simulink model "full_correlator"  (R2022a)
settings: Solver=VariableStepDiscrete  StartTime=0.0  StopTime=4000  RelTol=1e-3
libraries: hdlBasic x2638, hdlSSR x215, hdlDSPIP x4, xbsIndex_r4 x1, xps_library x1
(part 6 of 43)

== system full_correlator/Subsystem2/shared_bram3 ==
  addr : Inport
  data_in : Inport  Port=2
  we : Inport  Port=3
  Terminator : Terminator
  Terminator1 : Terminator
  Terminator2 : Terminator
  calc_add : Subsystem  mask{data_width=128, addr_width=6, sample_rate=sample_rate}
      mask prompts: data_width "data width"; addr_width "address width"; sample_rate "sample rate"
  convert_addr : hdlBasic/Convert  gui_display_data_type=Fixed-point  arith_type=Unsigned  n_bits=addr_width  bin_pt=0  float_type=Single  exp_bits=8  fraction_bits=24  quantization=Truncate  overflow=Wrap  en=off  latency=0  pipeline=off  XmcBlockStatus=1  maskContainerNames=group2  block_type=convert  block_config=sysgen:Convert_config  block_width=595  block_height=885
  convert_din1 : hdlBasic/Convert  gui_display_data_type=Fixed-point  arith_type=Unsigned  n_bits=128  bin_pt=0  float_type=Single  exp_bits=8  fraction_bits=24  quantization=Truncate  overflow=Wrap  en=off  latency=0  pipeline=off  XmcBlockStatus=1  maskContainerNames=group2  block_type=convert  block_config=sysgen:Convert_config  block_width=595  block_height=885
  convert_we : hdlBasic/Convert  gui_display_data_type=Fixed-point  arith_type=Unsigned  n_bits=1  bin_pt=0  float_type=Single  exp_bits=8  fraction_bits=24  quantization=Truncate  overflow=Wrap  en=off  latency=0  pipeline=off  XmcBlockStatus=1  maskContainerNames=group2  block_type=convert  block_config=sysgen:Convert_config  block_width=595  block_height=885
  full_correlator_Subsystem2_shared_bram3_addr : hdlBasic/Gateway Out  inherit_from_input=off  hdl_port=on  rows=1  columns=1  UseAsDAC=off  DACChannel='1'  interface=None  automatic_assignment=on  address_offset=hex2dec('00')  intf_name=''  intf_description=''  timing_constraint=None  locs_specified=off  LOCs={'A5','B9','A9','C1','A3','G6','E9','A6','A7','A8','B8','B1','B3','D9','B5','B4','B6','C2'}  io_standard={}  XmcBlockStatus=1  maskContainerNames=group4  block_type=gatewayout  block_config=sysgen:gateway_out_config  block_width_w=590  block_height_w=620  block_width=620  block_height=750
      settings: sginterface={'Nallatech'=>{'xdspkit'=>{'non_memory_mapped_port'=>'uprev_Shared_BRAM_addr'}},'Xilinx'=>{'jtaghwcosim'=>{'non_memory_mapped_port'=>'uprev_Shared_BRAM_addr'},'xdspkit'=>{'non_memory_mapped_port'=>'uprev_Shared_BRAM_addr'}}}
  full_correlator_Subsystem2_shared_bram3_data_in : hdlBasic/Gateway Out  inherit_from_input=off  hdl_port=on  rows=1  columns=1  UseAsDAC=off  DACChannel='1'  interface=None  automatic_assignment=on  address_offset=hex2dec('00')  intf_name=''  intf_description=''  timing_constraint=None  locs_specified=off  LOCs={'B21','B22','A22','B23','B19','C19','A20','A21','A23','B24','A24','A25','E18','D18','C18','B18'}  io_standard={}  XmcBlockStatus=1  maskContainerNames=group4  block_type=gatewayout  block_config=sysgen:gateway_out_config  block_width_w=590  block_height_w=620  block_width=620  block_height=750
      settings: sginterface={'Nallatech'=>{'xdspkit'=>{'non_memory_mapped_port'=>'uprev_Shared_BRAM_data_in'}},'Xilinx'=>{'jtaghwcosim'=>{'non_memory_mapped_port'=>'uprev_Shared_BRAM_data_in'},'xdspkit'=>{'non_memory_mapped_port'=>'uprev_Shared_BRAM_data_in'}}}
  full_correlator_Subsystem2_shared_bram3_data_out : hdlBasic/Gateway In  gui_display_data_type=Fixed-point  arith_type=Unsigned  n_bits=128  bin_pt=0  preci_type=Single  exp_width=8  frac_width=24  rows=1  columns=1  quantization=Truncate  overflow=Wrap  period=sample_rate  UseAsADC=off  ADCChannel='1'  interface=None  automatic_assignment=on  address_offset=hex2dec('00')  intf_name=''  intf_description=''  default_value=0  timing_constraint=None  locs_specified=off  LOCs={}  io_standard={}  inherit_from_input=off  hdl_port=on  XmcBlockStatus=1  maskContainerNames=group4  block_type=gatewayin  block_config=sysgen:gateway_in_config  block_width_w=590  block_height_w=620  block_width=640  block_height=850
      settings: sginterface={'Nallatech'=>{'xdspkit'=>{'non_memory_mapped_port'=>'uprev_Shared_BRAM_data_out'}},'Xilinx'=>{'jtaghwcosim'=>{'non_memory_mapped_port'=>'uprev_Shared_BRAM_data_out'},'xdspkit'=>{'non_memory_mapped_port'=>'uprev_Shared_BRAM_data_out'}}}
  full_correlator_Subsystem2_shared_bram3_we : hdlBasic/Gateway Out  inherit_from_input=off  hdl_port=on  rows=1  columns=1  UseAsDAC=off  DACChannel='1'  interface=None  automatic_assignment=on  address_offset=hex2dec('00')  intf_name=''  intf_description=''  timing_constraint=None  locs_specified=off  LOCs={'A14'}  io_standard={}  XmcBlockStatus=1  maskContainerNames=group4  block_type=gatewayout  block_config=sysgen:gateway_out_config  block_width_w=590  block_height_w=620  block_width=620  block_height=750
  munge_in : Subsystem  AncestorBlock=casper_library_flow_control/munge  mask(munge){divisions=4, div_size=[32 32 32 32], order=[3  2  1  0], arith_type_out=Unsigned, bin_pt_out=0}
      mask prompts: divisions "Number of divisions"; div_size "Division size (bits)"; order "Division packing order"; arith_type_out "Output arithmetic type"; bin_pt_out "Output binary point"
      mask help: Splits an input bus into the specified number of divisions and then recombines them in the order specified (most significant division = 0,least = number divisions-1)
      mask init:
      | munge_init(gcb, ...
      |     'divisions', divisions, ...
      |     'div_size', div_size, ...
      |     'order', order, ...
      |     'arith_type_out', arith_type_out, ...
      |     'bin_pt_out', bin_pt_out);
      settings: AttributesFormatString=|
      | split:[32 32 32 32]
      | join:[3 2 1 0]
      | Unsigned [128,0]
      mask TypeOptions arith_type_out: Unsigned | Signed  (2's comp) | Floating-point
  munge_out : Subsystem  AncestorBlock=casper_library_flow_control/munge  mask(munge){divisions=4, div_size=[32 32 32 32], order=[3  2  1  0], arith_type_out=Unsigned, bin_pt_out=0}
      mask prompts: divisions "Number of divisions"; div_size "Division size (bits)"; order "Division packing order"; arith_type_out "Output arithmetic type"; bin_pt_out "Output binary point"
      mask help: Splits an input bus into the specified number of divisions and then recombines them in the order specified (most significant division = 0,least = number divisions-1)
      mask init:
      | munge_init(gcb, ...
      |     'divisions', divisions, ...
      |     'div_size', div_size, ...
      |     'order', order, ...
      |     'arith_type_out', arith_type_out, ...
      |     'bin_pt_out', bin_pt_out);
      settings: AttributesFormatString=|
      | split:[32 32 32 32]
      | join:[3 2 1 0]
      | Unsigned [128,0]
      mask TypeOptions arith_type_out: Unsigned | Signed  (2's comp) | Floating-point
  sim_mem : Subsystem  mask{arith_type=Unsigned, addr_width=6, data_width=128, data_bin_pt=0, init_vals=[0   1   2   3   4   5   6   7   8   9  10  11  12  13  14  15  16  17  18  19  20  21  22  23  24  25  26  27  28  29  30  31  32  33  34  35  36  37  38  39  40  41  42  43  44  45  46  47  48  49  50  51  52  53  54  55  56  57  58  59  60  61  62  63], sample_rate=1, csp_latency=1}
      mask prompts: arith_type "Output Data Type"; addr_width "Address width"; data_width "Data width"; data_bin_pt "Data Binary Point"; init_vals "Initial values"; sample_rate "Sample rate"; csp_latency "Latency"
      mask init:
      | % set_param([gcb, '/data_to_xilinx'], 'arith_type', arith_type)
      | % set_param([gcb, '/data_to_xilinx'], 'n_bits', get_param(gcb, 'data_width'))
      mask TypeOptions arith_type: Unsigned | Signed  (2's comp)
      mask TypeOptions data_width: 8 | 16 | 32 | 64 | 128
  data_out : Outport  VectorParamsAs1DForOutWhenUnconnected=off
  wires:
  munge_out/1(dout) -> data_out/1
  sim_mem/1(data_out) -> full_correlator_Subsystem2_shared_bram3_data_out/1
  full_correlator_Subsystem2_shared_bram3_data_out/1 -> munge_out/1(din)
  convert_addr/1 -> full_correlator_Subsystem2_shared_bram3_addr/1
  convert_din1/1 -> full_correlator_Subsystem2_shared_bram3_data_in/1
  data_in/1 -> munge_in/1(din)
  calc_add/1(out) -> convert_addr/1
  full_correlator_Subsystem2_shared_bram3_we/1 -> Terminator2/1
  full_correlator_Subsystem2_shared_bram3_data_in/1 -> Terminator1/1
  full_correlator_Subsystem2_shared_bram3_addr/1 -> Terminator/1
  convert_we/1 -> full_correlator_Subsystem2_shared_bram3_we/1
  addr/1 -> sim_mem/1(addr), calc_add/1(in)
  we/1 -> sim_mem/3(we), convert_we/1
  munge_in/1(dout) -> sim_mem/2(data), convert_din1/1

== system full_correlator/Subsystem5/Subsystem ==
  din : Inport
  hold : Inport  Port=2
  Concat : hdlBasic/Concat  num_inputs=2  XmcBlockStatus=1  maskContainerNames=group1  block_type=concat  block_config=sysgen:Concat_config
  Scalar to Vector : hdlSSR/Scalar2Vector  Width=18  sg_ssr=16  block_type=scalar2vector_ssr  XmcBlockStatus=1  sg_ssr_prev=16  maskContainerNames=group1
  Vector Register : hdlSSR/Vector Register  init=[0, 0, 0, 0, 0,0,0,0]  rst=off  en=on  sg_ssr=8  block_type=register_ssr  XmcBlockStatus=1  sg_ssr_prev=8  maskContainerNames=group2
  Vector Reinterpret : hdlSSR/Vector Reinterpret  force_arith_type=on  arith_type="Signed  (2's comp)"  force_bin_pt=on  bin_pt=17  sg_ssr=16  block_type=reinterpret_ssr  XmcBlockStatus=1  sg_ssr_prev=16  maskContainerNames=group1
  Vector Reinterpret1 : hdlSSR/Vector Reinterpret  force_arith_type=on  arith_type=Unsigned  force_bin_pt=on  bin_pt=0  sg_ssr=8  block_type=reinterpret_ssr  XmcBlockStatus=1  sg_ssr_prev=8  maskContainerNames=group1
  Vector Reinterpret2 : hdlSSR/Vector Reinterpret  force_arith_type=on  arith_type=Unsigned  force_bin_pt=on  bin_pt=0  sg_ssr=8  block_type=reinterpret_ssr  XmcBlockStatus=1  sg_ssr_prev=8  maskContainerNames=group1
  Vector to Scalar : hdlSSR/Vector2Scalar  sg_ssr=8  block_type=vector2scalar_ssr  XmcBlockStatus=1  sg_ssr_prev=8  maskContainerNames=group1
  Vector to Scalar1 : hdlSSR/Vector2Scalar  sg_ssr=8  block_type=vector2scalar_ssr  XmcBlockStatus=1  sg_ssr_prev=8  maskContainerNames=group1
  out : Outport
  wires:
  Vector Reinterpret2/1 -> Vector to Scalar1/1
  Vector to Scalar/1 -> Concat/1
  Vector Reinterpret1/1 -> Vector to Scalar/1
  hold/1 -> Vector Register/2
  Vector Register/1 -> Vector Reinterpret2/1
  din/1 -> Vector Reinterpret1/1, Vector Register/1
  Scalar to Vector/1 -> Vector Reinterpret/1
  Concat/1 -> Scalar to Vector/1
  Vector Reinterpret/1 -> out/1
  Vector to Scalar1/1 -> Concat/2

== system full_correlator/Subsystem5/Subsystem1 ==
  din : Inport
  hold : Inport  Port=2
  Concat : hdlBasic/Concat  num_inputs=2  XmcBlockStatus=1  maskContainerNames=group1  block_type=concat  block_config=sysgen:Concat_config
  Scalar to Vector : hdlSSR/Scalar2Vector  Width=18  sg_ssr=16  block_type=scalar2vector_ssr  XmcBlockStatus=1  sg_ssr_prev=16  maskContainerNames=group1
  Vector Register : hdlSSR/Vector Register  init=[0, 0, 0, 0, 0,0,0,0]  rst=off  en=on  sg_ssr=8  block_type=register_ssr  XmcBlockStatus=1  sg_ssr_prev=8  maskContainerNames=group2
  Vector Reinterpret : hdlSSR/Vector Reinterpret  force_arith_type=on  arith_type="Signed  (2's comp)"  force_bin_pt=on  bin_pt=17  sg_ssr=16  block_type=reinterpret_ssr  XmcBlockStatus=1  sg_ssr_prev=16  maskContainerNames=group1
  Vector Reinterpret1 : hdlSSR/Vector Reinterpret  force_arith_type=on  arith_type=Unsigned  force_bin_pt=on  bin_pt=0  sg_ssr=8  block_type=reinterpret_ssr  XmcBlockStatus=1  sg_ssr_prev=8  maskContainerNames=group1
  Vector Reinterpret2 : hdlSSR/Vector Reinterpret  force_arith_type=on  arith_type=Unsigned  force_bin_pt=on  bin_pt=0  sg_ssr=8  block_type=reinterpret_ssr  XmcBlockStatus=1  sg_ssr_prev=8  maskContainerNames=group1
  Vector to Scalar : hdlSSR/Vector2Scalar  sg_ssr=8  block_type=vector2scalar_ssr  XmcBlockStatus=1  sg_ssr_prev=8  maskContainerNames=group1
  Vector to Scalar1 : hdlSSR/Vector2Scalar  sg_ssr=8  block_type=vector2scalar_ssr  XmcBlockStatus=1  sg_ssr_prev=8  maskContainerNames=group1
  out : Outport
  wires:
  Vector Reinterpret2/1 -> Vector to Scalar1/1
  Vector to Scalar/1 -> Concat/1
  Vector Reinterpret1/1 -> Vector to Scalar/1
  hold/1 -> Vector Register/2
  Vector Register/1 -> Vector Reinterpret2/1
  din/1 -> Vector Reinterpret1/1, Vector Register/1
  Scalar to Vector/1 -> Vector Reinterpret/1
  Concat/1 -> Scalar to Vector/1
  Vector Reinterpret/1 -> out/1
  Vector to Scalar1/1 -> Concat/2

== system full_correlator/Subsystem5/Subsystem2 ==
  w_addr : Inport
  d : Inport  Port=2
  we : Inport  Port=3
  addr_r : Inport  Port=4
  Constant4 : hdlBasic/Constant  const=127  gui_display_data_type=Fixed-point  arith_type=Unsigned  n_bits=7  bin_pt=0  preci_type=Single  exp_width=8  frac_width=24  explicit_period=on  period=1  XmcBlockStatus=1  maskContainerNames=tabcontainer1  block_type=constant  block_config=sysgen:Constant_config
  Convert : hdlBasic/Convert  gui_display_data_type=Fixed-point  arith_type=Unsigned  n_bits=1  bin_pt=0  float_type=Single  exp_bits=8  fraction_bits=24  quantization=Truncate  overflow=Wrap  en=off  latency=1  pipeline=off  XmcBlockStatus=1  maskContainerNames=group2  block_type=convert  block_config=sysgen:Convert_config  block_width=595  block_height=885
  Counter2 : hdlBasic/Counter  cnt_type=Free running  cnt_to=Inf  operation=Up  start_count=0  cnt_by_val=1  arith_type=Unsigned  n_bits=8  bin_pt=0  load_pin=off  rst=off  en=on  explicit_period=Explicit  period=1  use_behavioral_HDL=off  implementation=Fabric  XmcBlockStatus=1  maskContainerNames=group1  block_type=counter  block_config=sysgen:Counter_config  block_width=531  block_height=1023
  Delay : hdlBasic/Delay  rst=off  en=off  latency=1  reg_retiming=off  XmcBlockStatus=1  maskContainerNames=group1  block_type=delay  block_config=sysgen:Delay_config
  Delay2 : hdlBasic/Delay  rst=off  en=off  latency=2  reg_retiming=off  XmcBlockStatus=1  maskContainerNames=group1  block_type=delay  block_config=sysgen:Delay_config
  Delay3 : hdlBasic/Delay  rst=off  en=off  latency=1  reg_retiming=off  XmcBlockStatus=1  maskContainerNames=group1  block_type=delay  block_config=sysgen:Delay_config
  Inverter : hdlBasic/Inverter  en=off  latency=1  XmcBlockStatus=1  maskContainerNames=group2  block_type=inv  block_config=sysgen:Inverter_config
  Relational2 : hdlBasic/Relational  mode=a>b  op_type=Bool  en=off  latency=1  XmcBlockStatus=1  maskContainerNames=tabcontainer1  block_type=relational  block_config=sysgen:Relational_config
  Subsystem1 : Subsystem
  Subsystem2 : Subsystem
  Vector Delay : hdlSSR/Vector Delay  rst=off  en=off  vectorize_en=off  sg_latency=2  sg_ssr=16  reg_retiming=off  block_type=delay_ssr  XmcBlockStatus=1  sg_ssr_prev=16  maskContainerNames=group1
  Vector Mux{,1..3} (4 alike) : hdlSSR/Vector Mux  inputs=2  en=off  vectorize_en=off  vectorize_sel=off  sg_latency=1  sg_ssr=16  precision=Full  arith_type=Unsigned  n_bits=16  bin_pt=14  quantization=Truncate  overflow=Wrap  block_type=mux_ssr  inputs_prev=2  XmcBlockStatus=1  sg_ssr_prev=16  maskContainerNames=group1
  out_A : Outport
  out_B : Outport  Port=2
  out_C : Outport  Port=3
  out_D : Outport  Port=4
  wires:
  Counter2/1 -> Relational2/1
  Convert/1 -> Vector Mux/1, Vector Mux3/1, Vector Mux2/1, Vector Mux1/1
  Subsystem1/1(d_out_a) -> Vector Mux/3
  Subsystem2/2(d_out_b) -> Vector Mux1/2
  w_addr/1 -> Delay2/1
  d/1 -> Vector Delay/1
  Subsystem1/3(d_out_c) -> Vector Mux2/3
  addr_r/1 -> Delay3/1
  Subsystem2/4(d_out_d) -> Vector Mux3/2
  Constant4/1 -> Relational2/2
  Relational2/1 -> Inverter/1, Delay/1
  Delay/1 -> Subsystem1/3(we)
  Subsystem1/4(d_out_d) -> Vector Mux3/3
  Delay3/1 -> Subsystem1/7(addr_r_d), Subsystem1/6(addr_r_c), Subsystem1/5(addr_r_b), Subsystem1/4(addr_r_a), Subsystem2/7(addr_r_d), Subsystem2/6(addr_r_c), Subsystem2/5(addr_r_b), Subsystem2/4(addr_r_a)
  we/1 -> Counter2/1
  Delay2/1 -> Subsystem1/1(w_addr), Subsystem2/1(w_addr)
  Subsystem2/1(d_out_a) -> Vector Mux/2
  Subsystem1/2(d_out_b) -> Vector Mux1/3
  Vector Delay/1 -> Subsystem1/2(d_in), Subsystem2/2(d_in)
  Subsystem2/3(d_out_c) -> Vector Mux2/2
  Inverter/1 -> Convert/1, Subsystem2/3(we)
  Vector Mux/1 -> out_A/1
  Vector Mux1/1 -> out_B/1
  Vector Mux2/1 -> out_C/1
  Vector Mux3/1 -> out_D/1

== system full_correlator/Subsystem5/Subsystem3 ==
  we : Inport
  addr_w : Inport  Port=2
  addr_r : Inport  Port=3
  d : Inport  Port=4
  d1 : Inport  Port=5
  d2 : Inport  Port=6
  d3 : Inport  Port=7
  Constant6 : hdlBasic/Constant  const=127  gui_display_data_type=Fixed-point  arith_type=Unsigned  n_bits=7  bin_pt=0  preci_type=Single  exp_width=8  frac_width=24  explicit_period=on  period=1  XmcBlockStatus=1  maskContainerNames=tabcontainer1  block_type=constant  block_config=sysgen:Constant_config
  Convert1 : hdlBasic/Convert  gui_display_data_type=Fixed-point  arith_type=Unsigned  n_bits=1  bin_pt=0  float_type=Single  exp_bits=8  fraction_bits=24  quantization=Truncate  overflow=Wrap  en=off  latency=1  pipeline=off  XmcBlockStatus=1  maskContainerNames=group2  block_type=convert  block_config=sysgen:Convert_config  block_width=595  block_height=885
  Counter5 : hdlBasic/Counter  cnt_type=Free running  cnt_to=Inf  operation=Up  start_count=0  cnt_by_val=1  arith_type=Unsigned  n_bits=8  bin_pt=0  load_pin=off  rst=off  en=on  explicit_period=Explicit  period=1  use_behavioral_HDL=off  implementation=Fabric  XmcBlockStatus=1  maskContainerNames=group1  block_type=counter  block_config=sysgen:Counter_config  block_width=531  block_height=1023
  Delay1 : hdlBasic/Delay  rst=off  en=off  latency=1  reg_retiming=off  XmcBlockStatus=1  maskContainerNames=group1  block_type=delay  block_config=sysgen:Delay_config
  Delay2 : hdlBasic/Delay  rst=off  en=off  latency=2  reg_retiming=off  XmcBlockStatus=1  maskContainerNames=group1  block_type=delay  block_config=sysgen:Delay_config
  Delay3 : hdlBasic/Delay  rst=off  en=off  latency=3  reg_retiming=off  XmcBlockStatus=1  maskContainerNames=group1  block_type=delay  block_config=sysgen:Delay_config
  Inverter : hdlBasic/Inverter  en=off  latency=1  XmcBlockStatus=1  maskContainerNames=group2  block_type=inv  block_config=sysgen:Inverter_config
  Relational4 : hdlBasic/Relational  mode=a>b  op_type=Bool  en=off  latency=1  XmcBlockStatus=1  maskContainerNames=tabcontainer1  block_type=relational  block_config=sysgen:Relational_config
  Subsystem1 : Subsystem
  Subsystem3 : Subsystem
  Vector Delay{8..11} (4 alike) : hdlSSR/Vector Delay  rst=off  en=off  vectorize_en=off  sg_latency=2  sg_ssr=16  reg_retiming=off  block_type=delay_ssr  XmcBlockStatus=1  sg_ssr_prev=16  maskContainerNames=group1
  Vector Mux : hdlSSR/Vector Mux  inputs=2  en=off  vectorize_en=off  vectorize_sel=off  sg_latency=1  sg_ssr=16  precision=Full  arith_type=Unsigned  n_bits=16  bin_pt=14  quantization=Truncate  overflow=Wrap  block_type=mux_ssr  inputs_prev=2  XmcBlockStatus=1  sg_ssr_prev=16  maskContainerNames=group1
  out : Outport
  wires:
  Delay3/1 -> Subsystem1/1(addr_r), Subsystem3/1(addr_r)
  Constant6/1 -> Relational4/2
  Convert1/1 -> Vector Mux/1
  Subsystem1/1(out) -> Vector Mux/3
  Counter5/1 -> Relational4/1
  Subsystem3/1(out) -> Vector Mux/2
  Delay2/1 -> Subsystem1/2(addr_w), Subsystem3/2(addr_w)
  we/1 -> Counter5/1
  d/1 -> Vector Delay8/1
  d1/1 -> Vector Delay9/1
  Relational4/1 -> Inverter/1, Delay1/1
  Vector Mux/1 -> out/1
  Delay1/1 -> Subsystem1/3(we)
  d3/1 -> Vector Delay11/1
  Vector Delay11/1 -> Subsystem1/7(d_ind), Subsystem3/7(d_ind)
  addr_r/1 -> Delay3/1
  addr_w/1 -> Delay2/1
  d2/1 -> Vector Delay10/1
  Vector Delay8/1 -> Subsystem1/4(d_ina), Subsystem3/4(d_ina)
  Inverter/1 -> Convert1/1, Subsystem3/3(we)
  Vector Delay9/1 -> Subsystem1/5(d_inb), Subsystem3/5(d_inb)
  Vector Delay10/1 -> Subsystem1/6(d_inc), Subsystem3/6(d_inc)

== system full_correlator/Subsystem5/Subsystem4 ==
  w_addr : Inport
  d : Inport  Port=2
  we : Inport  Port=3
  addr_r : Inport  Port=4
  Constant4 : hdlBasic/Constant  const=127  gui_display_data_type=Fixed-point  arith_type=Unsigned  n_bits=7  bin_pt=0  preci_type=Single  exp_width=8  frac_width=24  explicit_period=on  period=1  XmcBlockStatus=1  maskContainerNames=tabcontainer1  block_type=constant  block_config=sysgen:Constant_config
  Convert : hdlBasic/Convert  gui_display_data_type=Fixed-point  arith_type=Unsigned  n_bits=1  bin_pt=0  float_type=Single  exp_bits=8  fraction_bits=24  quantization=Truncate  overflow=Wrap  en=off  latency=1  pipeline=off  XmcBlockStatus=1  maskContainerNames=group2  block_type=convert  block_config=sysgen:Convert_config  block_width=595  block_height=885
  Counter2 : hdlBasic/Counter  cnt_type=Free running  cnt_to=Inf  operation=Up  start_count=0  cnt_by_val=1  arith_type=Unsigned  n_bits=8  bin_pt=0  load_pin=off  rst=off  en=on  explicit_period=Explicit  period=1  use_behavioral_HDL=off  implementation=Fabric  XmcBlockStatus=1  maskContainerNames=group1  block_type=counter  block_config=sysgen:Counter_config  block_width=531  block_height=1023
  Delay : hdlBasic/Delay  rst=off  en=off  latency=1  reg_retiming=off  XmcBlockStatus=1  maskContainerNames=group1  block_type=delay  block_config=sysgen:Delay_config
  Delay2 : hdlBasic/Delay  rst=off  en=off  latency=2  reg_retiming=off  XmcBlockStatus=1  maskContainerNames=group1  block_type=delay  block_config=sysgen:Delay_config
  Delay3 : hdlBasic/Delay  rst=off  en=off  latency=1  reg_retiming=off  XmcBlockStatus=1  maskContainerNames=group1  block_type=delay  block_config=sysgen:Delay_config
  Inverter : hdlBasic/Inverter  en=off  latency=1  XmcBlockStatus=1  maskContainerNames=group2  block_type=inv  block_config=sysgen:Inverter_config
  Relational2 : hdlBasic/Relational  mode=a>b  op_type=Bool  en=off  latency=1  XmcBlockStatus=1  maskContainerNames=tabcontainer1  block_type=relational  block_config=sysgen:Relational_config
  Subsystem1 : Subsystem
  Subsystem2 : Subsystem
  Vector Delay : hdlSSR/Vector Delay  rst=off  en=off  vectorize_en=off  sg_latency=2  sg_ssr=16  reg_retiming=off  block_type=delay_ssr  XmcBlockStatus=1  sg_ssr_prev=16  maskContainerNames=group1
  Vector Mux{,1..3} (4 alike) : hdlSSR/Vector Mux  inputs=2  en=off  vectorize_en=off  vectorize_sel=off  sg_latency=1  sg_ssr=16  precision=Full  arith_type=Unsigned  n_bits=16  bin_pt=14  quantization=Truncate  overflow=Wrap  block_type=mux_ssr  inputs_prev=2  XmcBlockStatus=1  sg_ssr_prev=16  maskContainerNames=group1
  out_A : Outport
  out_B : Outport  Port=2
  out_C : Outport  Port=3
  out_D : Outport  Port=4
  wires:
  Counter2/1 -> Relational2/1
  Convert/1 -> Vector Mux/1, Vector Mux3/1, Vector Mux2/1, Vector Mux1/1
  Subsystem1/1(d_out_a) -> Vector Mux/3
  Subsystem2/2(d_out_b) -> Vector Mux1/2
  w_addr/1 -> Delay2/1
  d/1 -> Vector Delay/1
  Subsystem1/3(d_out_c) -> Vector Mux2/3
  addr_r/1 -> Delay3/1
  Subsystem2/4(d_out_d) -> Vector Mux3/2
  Constant4/1 -> Relational2/2
  Relational2/1 -> Inverter/1, Delay/1
  Delay/1 -> Subsystem1/3(we)
  Subsystem1/4(d_out_d) -> Vector Mux3/3
  Delay3/1 -> Subsystem1/7(addr_r_d), Subsystem1/6(addr_r_c), Subsystem1/5(addr_r_b), Subsystem1/4(addr_r_a), Subsystem2/7(addr_r_d), Subsystem2/6(addr_r_c), Subsystem2/5(addr_r_b), Subsystem2/4(addr_r_a)
  we/1 -> Counter2/1
  Delay2/1 -> Subsystem1/1(w_addr), Subsystem2/1(w_addr)
  Subsystem2/1(d_out_a) -> Vector Mux/2
  Subsystem1/2(d_out_b) -> Vector Mux1/3
  Vector Delay/1 -> Subsystem1/2(d_in), Subsystem2/2(d_in)
  Subsystem2/3(d_out_c) -> Vector Mux2/2
  Inverter/1 -> Convert/1, Subsystem2/3(we)
  Vector Mux/1 -> out_A/1
  Vector Mux1/1 -> out_B/1
  Vector Mux2/1 -> out_C/1
  Vector Mux3/1 -> out_D/1

== system full_correlator/Subsystem5/Subsystem5 ==
  we : Inport
  addr_w : Inport  Port=2
  addr_r : Inport  Port=3
  d : Inport  Port=4
  d1 : Inport  Port=5
  d2 : Inport  Port=6
  d3 : Inport  Port=7
  Constant6 : hdlBasic/Constant  const=127  gui_display_data_type=Fixed-point  arith_type=Unsigned  n_bits=7  bin_pt=0  preci_type=Single  exp_width=8  frac_width=24  explicit_period=on  period=1  XmcBlockStatus=1  maskContainerNames=tabcontainer1  block_type=constant  block_config=sysgen:Constant_config
  Convert1 : hdlBasic/Convert  gui_display_data_type=Fixed-point  arith_type=Unsigned  n_bits=1  bin_pt=0  float_type=Single  exp_bits=8  fraction_bits=24  quantization=Truncate  overflow=Wrap  en=off  latency=1  pipeline=off  XmcBlockStatus=1  maskContainerNames=group2  block_type=convert  block_config=sysgen:Convert_config  block_width=595  block_height=885
  Counter5 : hdlBasic/Counter  cnt_type=Free running  cnt_to=Inf  operation=Up  start_count=0  cnt_by_val=1  arith_type=Unsigned  n_bits=8  bin_pt=0  load_pin=off  rst=off  en=on  explicit_period=Explicit  period=1  use_behavioral_HDL=off  implementation=Fabric  XmcBlockStatus=1  maskContainerNames=group1  block_type=counter  block_config=sysgen:Counter_config  block_width=531  block_height=1023
  Delay1 : hdlBasic/Delay  rst=off  en=off  latency=1  reg_retiming=off  XmcBlockStatus=1  maskContainerNames=group1  block_type=delay  block_config=sysgen:Delay_config
  Delay2 : hdlBasic/Delay  rst=off  en=off  latency=2  reg_retiming=off  XmcBlockStatus=1  maskContainerNames=group1  block_type=delay  block_config=sysgen:Delay_config
  Delay3 : hdlBasic/Delay  rst=off  en=off  latency=3  reg_retiming=off  XmcBlockStatus=1  maskContainerNames=group1  block_type=delay  block_config=sysgen:Delay_config
  Inverter : hdlBasic/Inverter  en=off  latency=1  XmcBlockStatus=1  maskContainerNames=group2  block_type=inv  block_config=sysgen:Inverter_config
  Relational4 : hdlBasic/Relational  mode=a>b  op_type=Bool  en=off  latency=1  XmcBlockStatus=1  maskContainerNames=tabcontainer1  block_type=relational  block_config=sysgen:Relational_config
  Subsystem1 : Subsystem
  Subsystem3 : Subsystem
  Vector Delay{8..11} (4 alike) : hdlSSR/Vector Delay  rst=off  en=off  vectorize_en=off  sg_latency=2  sg_ssr=16  reg_retiming=off  block_type=delay_ssr  XmcBlockStatus=1  sg_ssr_prev=16  maskContainerNames=group1
  Vector Mux : hdlSSR/Vector Mux  inputs=2  en=off  vectorize_en=off  vectorize_sel=off  sg_latency=1  sg_ssr=16  precision=Full  arith_type=Unsigned  n_bits=16  bin_pt=14  quantization=Truncate  overflow=Wrap  block_type=mux_ssr  inputs_prev=2  XmcBlockStatus=1  sg_ssr_prev=16  maskContainerNames=group1
  out : Outport
  wires:
  Delay3/1 -> Subsystem1/1(addr_r), Subsystem3/1(addr_r)
  Constant6/1 -> Relational4/2
  Convert1/1 -> Vector Mux/1
  Subsystem1/1(out) -> Vector Mux/3
  Counter5/1 -> Relational4/1
  Subsystem3/1(out) -> Vector Mux/2
  Delay2/1 -> Subsystem1/2(addr_w), Subsystem3/2(addr_w)
  we/1 -> Counter5/1
  d/1 -> Vector Delay8/1
  d1/1 -> Vector Delay9/1
  Relational4/1 -> Inverter/1, Delay1/1
  Vector Mux/1 -> out/1
  Delay1/1 -> Subsystem1/3(we)
  d3/1 -> Vector Delay11/1
  Vector Delay11/1 -> Subsystem1/7(d_ind), Subsystem3/7(d_ind)
  addr_r/1 -> Delay3/1
  addr_w/1 -> Delay2/1
  d2/1 -> Vector Delay10/1
  Vector Delay8/1 -> Subsystem1/4(d_ina), Subsystem3/4(d_ina)
  Inverter/1 -> Convert1/1, Subsystem3/3(we)
  Vector Delay9/1 -> Subsystem1/5(d_inb), Subsystem3/5(d_inb)
  Vector Delay10/1 -> Subsystem1/6(d_inc), Subsystem3/6(d_inc)

== system full_correlator/Subsystem5/Vector Complex Mult ==
  A_re : Inport
  A_im : Inport  Port=2
  B_re : Inport  Port=3
  B_im : Inport  Port=4
  DemuxAim : Demux  Outputs=16
  DemuxAre : Demux  Outputs=16
  DemuxBim : Demux  Outputs=16
  DemuxBre : Demux  Outputs=16
  Mult0 : Subsystem
  Mult1 : Subsystem
  Mult10 : Subsystem
  Mult11 : Subsystem
  Mult12 : Subsystem
  Mult13 : Subsystem
  Mult14 : Subsystem
  Mult15 : Subsystem
  Mult2 : Subsystem
  Mult3 : Subsystem
  Mult4 : Subsystem
  Mult5 : Subsystem
  Mult6 : Subsystem
  Mult7 : Subsystem
  Mult8 : Subsystem
  Mult9 : Subsystem
  MuxCim : Mux  Inputs=16
  MuxCre : Mux  Inputs=16
  C_re : Outport  VectorParamsAs1DForOutWhenUnconnected=off
  C_im : Outport  Port=2  VectorParamsAs1DForOutWhenUnconnected=off
  wires:
  Mult0/1(C_re) -> MuxCre/1
  Mult0/2(C_im) -> MuxCim/1
  Mult1/1(C_re) -> MuxCre/2
  Mult1/2(C_im) -> MuxCim/2
  Mult2/1(C_re) -> MuxCre/3
  Mult2/2(C_im) -> MuxCim/3
  Mult3/1(C_re) -> MuxCre/4
  Mult3/2(C_im) -> MuxCim/4
  Mult4/1(C_re) -> MuxCre/5
  Mult4/2(C_im) -> MuxCim/5
  Mult5/1(C_re) -> MuxCre/6
  Mult5/2(C_im) -> MuxCim/6
  Mult6/1(C_re) -> MuxCre/7
  Mult6/2(C_im) -> MuxCim/7
  Mult7/1(C_re) -> MuxCre/8
  Mult7/2(C_im) -> MuxCim/8
  Mult8/1(C_re) -> MuxCre/9
  Mult8/2(C_im) -> MuxCim/9
  Mult9/1(C_re) -> MuxCre/10
  Mult9/2(C_im) -> MuxCim/10
  Mult10/1(C_re) -> MuxCre/11
  Mult10/2(C_im) -> MuxCim/11
  Mult11/1(C_re) -> MuxCre/12
  Mult11/2(C_im) -> MuxCim/12
  Mult12/1(C_re) -> MuxCre/13
  Mult12/2(C_im) -> MuxCim/13
  Mult13/1(C_re) -> MuxCre/14
  Mult13/2(C_im) -> MuxCim/14
  Mult14/1(C_re) -> MuxCre/15
  Mult14/2(C_im) -> MuxCim/15
  Mult15/1(C_re) -> MuxCre/16
  Mult15/2(C_im) -> MuxCim/16
  MuxCre/1 -> C_re/1
  MuxCim/1 -> C_im/1
  DemuxAre/1 -> Mult0/1(A_re)
  DemuxAim/1 -> Mult0/2(A_im)
  DemuxBre/1 -> Mult0/3(B_re)
  DemuxBim/1 -> Mult0/4(B_im)
  DemuxAre/2 -> Mult1/1(A_re)
  DemuxAim/2 -> Mult1/2(A_im)
  DemuxBre/2 -> Mult1/3(B_re)
  DemuxBim/2 -> Mult1/4(B_im)
  DemuxAre/3 -> Mult2/1(A_re)
  DemuxAim/3 -> Mult2/2(A_im)
  DemuxBre/3 -> Mult2/3(B_re)
  DemuxBim/3 -> Mult2/4(B_im)
  DemuxAre/4 -> Mult3/1(A_re)
  DemuxAim/4 -> Mult3/2(A_im)
  DemuxBre/4 -> Mult3/3(B_re)
  DemuxBim/4 -> Mult3/4(B_im)
  DemuxAre/5 -> Mult4/1(A_re)
  DemuxAim/5 -> Mult4/2(A_im)
  DemuxBre/5 -> Mult4/3(B_re)
  DemuxBim/5 -> Mult4/4(B_im)
  DemuxAre/6 -> Mult5/1(A_re)
  DemuxAim/6 -> Mult5/2(A_im)
  DemuxBre/6 -> Mult5/3(B_re)
  DemuxBim/6 -> Mult5/4(B_im)
  DemuxAre/7 -> Mult6/1(A_re)
  DemuxAim/7 -> Mult6/2(A_im)
  DemuxBre/7 -> Mult6/3(B_re)
  DemuxBim/7 -> Mult6/4(B_im)
  DemuxAre/8 -> Mult7/1(A_re)
  DemuxAim/8 -> Mult7/2(A_im)
  DemuxBre/8 -> Mult7/3(B_re)
  DemuxBim/8 -> Mult7/4(B_im)
  DemuxAre/9 -> Mult8/1(A_re)
  DemuxAim/9 -> Mult8/2(A_im)
  DemuxBre/9 -> Mult8/3(B_re)
  DemuxBim/9 -> Mult8/4(B_im)
  DemuxAre/10 -> Mult9/1(A_re)
  DemuxAim/10 -> Mult9/2(A_im)
  DemuxBre/10 -> Mult9/3(B_re)
  DemuxBim/10 -> Mult9/4(B_im)
  DemuxAre/11 -> Mult10/1(A_re)
  DemuxAim/11 -> Mult10/2(A_im)
  DemuxBre/11 -> Mult10/3(B_re)
  DemuxBim/11 -> Mult10/4(B_im)
  DemuxAre/12 -> Mult11/1(A_re)
  DemuxAim/12 -> Mult11/2(A_im)
  DemuxBre/12 -> Mult11/3(B_re)
  DemuxBim/12 -> Mult11/4(B_im)
  DemuxAre/13 -> Mult12/1(A_re)
  DemuxAim/13 -> Mult12/2(A_im)
  DemuxBre/13 -> Mult12/3(B_re)
  DemuxBim/13 -> Mult12/4(B_im)
  DemuxAre/14 -> Mult13/1(A_re)
  DemuxAim/14 -> Mult13/2(A_im)
  DemuxBre/14 -> Mult13/3(B_re)
  DemuxBim/14 -> Mult13/4(B_im)
  DemuxAre/15 -> Mult14/1(A_re)
  DemuxAim/15 -> Mult14/2(A_im)
  DemuxBre/15 -> Mult14/3(B_re)
  DemuxBim/15 -> Mult14/4(B_im)
  DemuxAre/16 -> Mult15/1(A_re)
  DemuxAim/16 -> Mult15/2(A_im)
  DemuxBre/16 -> Mult15/3(B_re)
  DemuxBim/16 -> Mult15/4(B_im)
  A_re/1 -> DemuxAre/1
  A_im/1 -> DemuxAim/1
  B_re/1 -> DemuxBre/1
  B_im/1 -> DemuxBim/1

== system full_correlator/Subsystem5/Vector Complex Mult1 ==
  A_re : Inport
  A_im : Inport  Port=2
  B_re : Inport  Port=3
  B_im : Inport  Port=4
  DemuxAim : Demux  Outputs=16
  DemuxAre : Demux  Outputs=16
  DemuxBim : Demux  Outputs=16
  DemuxBre : Demux  Outputs=16
  Mult0 : Subsystem
  Mult1 : Subsystem
  Mult10 : Subsystem
  Mult11 : Subsystem
  Mult12 : Subsystem
  Mult13 : Subsystem
  Mult14 : Subsystem
  Mult15 : Subsystem
  Mult2 : Subsystem
  Mult3 : Subsystem
  Mult4 : Subsystem
  Mult5 : Subsystem
  Mult6 : Subsystem
  Mult7 : Subsystem
  Mult8 : Subsystem
  Mult9 : Subsystem
  MuxCim : Mux  Inputs=16
  MuxCre : Mux  Inputs=16
  C_re : Outport  VectorParamsAs1DForOutWhenUnconnected=off
  C_im : Outport  Port=2  VectorParamsAs1DForOutWhenUnconnected=off
  wires:
  Mult0/1(C_re) -> MuxCre/1
  Mult0/2(C_im) -> MuxCim/1
  Mult1/1(C_re) -> MuxCre/2
  Mult1/2(C_im) -> MuxCim/2
  Mult2/1(C_re) -> MuxCre/3
  Mult2/2(C_im) -> MuxCim/3
  Mult3/1(C_re) -> MuxCre/4
  Mult3/2(C_im) -> MuxCim/4
  Mult4/1(C_re) -> MuxCre/5
  Mult4/2(C_im) -> MuxCim/5
  Mult5/1(C_re) -> MuxCre/6
  Mult5/2(C_im) -> MuxCim/6
  Mult6/1(C_re) -> MuxCre/7
  Mult6/2(C_im) -> MuxCim/7
  Mult7/1(C_re) -> MuxCre/8
  Mult7/2(C_im) -> MuxCim/8
  Mult8/1(C_re) -> MuxCre/9
  Mult8/2(C_im) -> MuxCim/9
  Mult9/1(C_re) -> MuxCre/10
  Mult9/2(C_im) -> MuxCim/10
  Mult10/1(C_re) -> MuxCre/11
  Mult10/2(C_im) -> MuxCim/11
  Mult11/1(C_re) -> MuxCre/12
  Mult11/2(C_im) -> MuxCim/12
  Mult12/1(C_re) -> MuxCre/13
  Mult12/2(C_im) -> MuxCim/13
  Mult13/1(C_re) -> MuxCre/14
  Mult13/2(C_im) -> MuxCim/14
  Mult14/1(C_re) -> MuxCre/15
  Mult14/2(C_im) -> MuxCim/15
  Mult15/1(C_re) -> MuxCre/16
  Mult15/2(C_im) -> MuxCim/16
  MuxCre/1 -> C_re/1
  MuxCim/1 -> C_im/1
  DemuxAre/1 -> Mult0/1(A_re)
  DemuxAim/1 -> Mult0/2(A_im)
  DemuxBre/1 -> Mult0/3(B_re)
  DemuxBim/1 -> Mult0/4(B_im)
  DemuxAre/2 -> Mult1/1(A_re)
  DemuxAim/2 -> Mult1/2(A_im)
  DemuxBre/2 -> Mult1/3(B_re)
  DemuxBim/2 -> Mult1/4(B_im)
  DemuxAre/3 -> Mult2/1(A_re)
  DemuxAim/3 -> Mult2/2(A_im)
  DemuxBre/3 -> Mult2/3(B_re)
  DemuxBim/3 -> Mult2/4(B_im)
  DemuxAre/4 -> Mult3/1(A_re)
  DemuxAim/4 -> Mult3/2(A_im)
  DemuxBre/4 -> Mult3/3(B_re)
  DemuxBim/4 -> Mult3/4(B_im)
  DemuxAre/5 -> Mult4/1(A_re)
  DemuxAim/5 -> Mult4/2(A_im)
  DemuxBre/5 -> Mult4/3(B_re)
  DemuxBim/5 -> Mult4/4(B_im)
  DemuxAre/6 -> Mult5/1(A_re)
  DemuxAim/6 -> Mult5/2(A_im)
  DemuxBre/6 -> Mult5/3(B_re)
  DemuxBim/6 -> Mult5/4(B_im)
  DemuxAre/7 -> Mult6/1(A_re)
  DemuxAim/7 -> Mult6/2(A_im)
  DemuxBre/7 -> Mult6/3(B_re)
  DemuxBim/7 -> Mult6/4(B_im)
  DemuxAre/8 -> Mult7/1(A_re)
  DemuxAim/8 -> Mult7/2(A_im)
  DemuxBre/8 -> Mult7/3(B_re)
  DemuxBim/8 -> Mult7/4(B_im)
  DemuxAre/9 -> Mult8/1(A_re)
  DemuxAim/9 -> Mult8/2(A_im)
  DemuxBre/9 -> Mult8/3(B_re)
  DemuxBim/9 -> Mult8/4(B_im)
  DemuxAre/10 -> Mult9/1(A_re)
  DemuxAim/10 -> Mult9/2(A_im)
  DemuxBre/10 -> Mult9/3(B_re)
  DemuxBim/10 -> Mult9/4(B_im)
  DemuxAre/11 -> Mult10/1(A_re)
  DemuxAim/11 -> Mult10/2(A_im)
  DemuxBre/11 -> Mult10/3(B_re)
  DemuxBim/11 -> Mult10/4(B_im)
  DemuxAre/12 -> Mult11/1(A_re)
  DemuxAim/12 -> Mult11/2(A_im)
  DemuxBre/12 -> Mult11/3(B_re)
  DemuxBim/12 -> Mult11/4(B_im)
  DemuxAre/13 -> Mult12/1(A_re)
  DemuxAim/13 -> Mult12/2(A_im)
  DemuxBre/13 -> Mult12/3(B_re)
  DemuxBim/13 -> Mult12/4(B_im)
  DemuxAre/14 -> Mult13/1(A_re)
  DemuxAim/14 -> Mult13/2(A_im)
  DemuxBre/14 -> Mult13/3(B_re)
  DemuxBim/14 -> Mult13/4(B_im)
  DemuxAre/15 -> Mult14/1(A_re)
  DemuxAim/15 -> Mult14/2(A_im)
  DemuxBre/15 -> Mult14/3(B_re)
  DemuxBim/15 -> Mult14/4(B_im)
  DemuxAre/16 -> Mult15/1(A_re)
  DemuxAim/16 -> Mult15/2(A_im)
  DemuxBre/16 -> Mult15/3(B_re)
  DemuxBim/16 -> Mult15/4(B_im)
  A_re/1 -> DemuxAre/1
  A_im/1 -> DemuxAim/1
  B_re/1 -> DemuxBre/1
  B_im/1 -> DemuxBim/1

== system full_correlator/Subsystem5/Vector Complex Mult2 ==
  A_re : Inport
  A_im : Inport  Port=2
  B_re : Inport  Port=3
  B_im : Inport  Port=4
  DemuxAim : Demux  Outputs=16
  DemuxAre : Demux  Outputs=16
  DemuxBim : Demux  Outputs=16
  DemuxBre : Demux  Outputs=16
  Mult0 : Subsystem
  Mult1 : Subsystem
  Mult10 : Subsystem
  Mult11 : Subsystem
  Mult12 : Subsystem
  Mult13 : Subsystem
  Mult14 : Subsystem
  Mult15 : Subsystem
  Mult2 : Subsystem
  Mult3 : Subsystem
  Mult4 : Subsystem
  Mult5 : Subsystem
  Mult6 : Subsystem
  Mult7 : Subsystem
  Mult8 : Subsystem
  Mult9 : Subsystem
  MuxCim : Mux  Inputs=16
  MuxCre : Mux  Inputs=16
  C_re : Outport  VectorParamsAs1DForOutWhenUnconnected=off
  C_im : Outport  Port=2  VectorParamsAs1DForOutWhenUnconnected=off
  wires:
  Mult0/1(C_re) -> MuxCre/1
  Mult0/2(C_im) -> MuxCim/1
  Mult1/1(C_re) -> MuxCre/2
  Mult1/2(C_im) -> MuxCim/2
  Mult2/1(C_re) -> MuxCre/3
  Mult2/2(C_im) -> MuxCim/3
  Mult3/1(C_re) -> MuxCre/4
  Mult3/2(C_im) -> MuxCim/4
  Mult4/1(C_re) -> MuxCre/5
  Mult4/2(C_im) -> MuxCim/5
  Mult5/1(C_re) -> MuxCre/6
  Mult5/2(C_im) -> MuxCim/6
  Mult6/1(C_re) -> MuxCre/7
  Mult6/2(C_im) -> MuxCim/7
  Mult7/1(C_re) -> MuxCre/8
  Mult7/2(C_im) -> MuxCim/8
  Mult8/1(C_re) -> MuxCre/9
  Mult8/2(C_im) -> MuxCim/9
  Mult9/1(C_re) -> MuxCre/10
  Mult9/2(C_im) -> MuxCim/10
  Mult10/1(C_re) -> MuxCre/11
  Mult10/2(C_im) -> MuxCim/11
  Mult11/1(C_re) -> MuxCre/12
  Mult11/2(C_im) -> MuxCim/12
  Mult12/1(C_re) -> MuxCre/13
  Mult12/2(C_im) -> MuxCim/13
  Mult13/1(C_re) -> MuxCre/14
  Mult13/2(C_im) -> MuxCim/14
  Mult14/1(C_re) -> MuxCre/15
  Mult14/2(C_im) -> MuxCim/15
  Mult15/1(C_re) -> MuxCre/16
  Mult15/2(C_im) -> MuxCim/16
  MuxCre/1 -> C_re/1
  MuxCim/1 -> C_im/1
  DemuxAre/1 -> Mult0/1(A_re)
  DemuxAim/1 -> Mult0/2(A_im)
  DemuxBre/1 -> Mult0/3(B_re)
  DemuxBim/1 -> Mult0/4(B_im)
  DemuxAre/2 -> Mult1/1(A_re)
  DemuxAim/2 -> Mult1/2(A_im)
  DemuxBre/2 -> Mult1/3(B_re)
  DemuxBim/2 -> Mult1/4(B_im)
  DemuxAre/3 -> Mult2/1(A_re)
  DemuxAim/3 -> Mult2/2(A_im)
  DemuxBre/3 -> Mult2/3(B_re)
  DemuxBim/3 -> Mult2/4(B_im)
  DemuxAre/4 -> Mult3/1(A_re)
  DemuxAim/4 -> Mult3/2(A_im)
  DemuxBre/4 -> Mult3/3(B_re)
  DemuxBim/4 -> Mult3/4(B_im)
  DemuxAre/5 -> Mult4/1(A_re)
  DemuxAim/5 -> Mult4/2(A_im)
  DemuxBre/5 -> Mult4/3(B_re)
  DemuxBim/5 -> Mult4/4(B_im)
  DemuxAre/6 -> Mult5/1(A_re)
  DemuxAim/6 -> Mult5/2(A_im)
  DemuxBre/6 -> Mult5/3(B_re)
  DemuxBim/6 -> Mult5/4(B_im)
  DemuxAre/7 -> Mult6/1(A_re)
  DemuxAim/7 -> Mult6/2(A_im)
  DemuxBre/7 -> Mult6/3(B_re)
  DemuxBim/7 -> Mult6/4(B_im)
  DemuxAre/8 -> Mult7/1(A_re)
  DemuxAim/8 -> Mult7/2(A_im)
  DemuxBre/8 -> Mult7/3(B_re)
  DemuxBim/8 -> Mult7/4(B_im)
  DemuxAre/9 -> Mult8/1(A_re)
  DemuxAim/9 -> Mult8/2(A_im)
  DemuxBre/9 -> Mult8/3(B_re)
  DemuxBim/9 -> Mult8/4(B_im)
  DemuxAre/10 -> Mult9/1(A_re)
  DemuxAim/10 -> Mult9/2(A_im)
  DemuxBre/10 -> Mult9/3(B_re)
  DemuxBim/10 -> Mult9/4(B_im)
  DemuxAre/11 -> Mult10/1(A_re)
  DemuxAim/11 -> Mult10/2(A_im)
  DemuxBre/11 -> Mult10/3(B_re)
  DemuxBim/11 -> Mult10/4(B_im)
  DemuxAre/12 -> Mult11/1(A_re)
  DemuxAim/12 -> Mult11/2(A_im)
  DemuxBre/12 -> Mult11/3(B_re)
  DemuxBim/12 -> Mult11/4(B_im)
  DemuxAre/13 -> Mult12/1(A_re)
  DemuxAim/13 -> Mult12/2(A_im)
  DemuxBre/13 -> Mult12/3(B_re)
  DemuxBim/13 -> Mult12/4(B_im)
  DemuxAre/14 -> Mult13/1(A_re)
  DemuxAim/14 -> Mult13/2(A_im)
  DemuxBre/14 -> Mult13/3(B_re)
  DemuxBim/14 -> Mult13/4(B_im)
  DemuxAre/15 -> Mult14/1(A_re)
  DemuxAim/15 -> Mult14/2(A_im)
  DemuxBre/15 -> Mult14/3(B_re)
  DemuxBim/15 -> Mult14/4(B_im)
  DemuxAre/16 -> Mult15/1(A_re)
  DemuxAim/16 -> Mult15/2(A_im)
  DemuxBre/16 -> Mult15/3(B_re)
  DemuxBim/16 -> Mult15/4(B_im)
  A_re/1 -> DemuxAre/1
  A_im/1 -> DemuxAim/1
  B_re/1 -> DemuxBre/1
  B_im/1 -> DemuxBim/1

== system full_correlator/Subsystem5/Vector Complex Mult3 ==
  A_re : Inport
  A_im : Inport  Port=2
  B_re : Inport  Port=3
  B_im : Inport  Port=4
  DemuxAim : Demux  Outputs=16
  DemuxAre : Demux  Outputs=16
  DemuxBim : Demux  Outputs=16
  DemuxBre : Demux  Outputs=16
  Mult0 : Subsystem
  Mult1 : Subsystem
  Mult10 : Subsystem
  Mult11 : Subsystem
  Mult12 : Subsystem
  Mult13 : Subsystem
  Mult14 : Subsystem
  Mult15 : Subsystem
  Mult2 : Subsystem
  Mult3 : Subsystem
  Mult4 : Subsystem
  Mult5 : Subsystem
  Mult6 : Subsystem
  Mult7 : Subsystem
  Mult8 : Subsystem
  Mult9 : Subsystem
  MuxCim : Mux  Inputs=16
  MuxCre : Mux  Inputs=16
  C_re : Outport  VectorParamsAs1DForOutWhenUnconnected=off
  C_im : Outport  Port=2  VectorParamsAs1DForOutWhenUnconnected=off
  wires:
  Mult0/1(C_re) -> MuxCre/1
  Mult0/2(C_im) -> MuxCim/1
  Mult1/1(C_re) -> MuxCre/2
  Mult1/2(C_im) -> MuxCim/2
  Mult2/1(C_re) -> MuxCre/3
  Mult2/2(C_im) -> MuxCim/3
  Mult3/1(C_re) -> MuxCre/4
  Mult3/2(C_im) -> MuxCim/4
  Mult4/1(C_re) -> MuxCre/5
  Mult4/2(C_im) -> MuxCim/5
  Mult5/1(C_re) -> MuxCre/6
  Mult5/2(C_im) -> MuxCim/6
  Mult6/1(C_re) -> MuxCre/7
  Mult6/2(C_im) -> MuxCim/7
  Mult7/1(C_re) -> MuxCre/8
  Mult7/2(C_im) -> MuxCim/8
  Mult8/1(C_re) -> MuxCre/9
  Mult8/2(C_im) -> MuxCim/9
  Mult9/1(C_re) -> MuxCre/10
  Mult9/2(C_im) -> MuxCim/10
  Mult10/1(C_re) -> MuxCre/11
  Mult10/2(C_im) -> MuxCim/11
  Mult11/1(C_re) -> MuxCre/12
  Mult11/2(C_im) -> MuxCim/12
  Mult12/1(C_re) -> MuxCre/13
  Mult12/2(C_im) -> MuxCim/13
  Mult13/1(C_re) -> MuxCre/14
  Mult13/2(C_im) -> MuxCim/14
  Mult14/1(C_re) -> MuxCre/15
  Mult14/2(C_im) -> MuxCim/15
  Mult15/1(C_re) -> MuxCre/16
  Mult15/2(C_im) -> MuxCim/16
  MuxCre/1 -> C_re/1
  MuxCim/1 -> C_im/1
  DemuxAre/1 -> Mult0/1(A_re)
  DemuxAim/1 -> Mult0/2(A_im)
  DemuxBre/1 -> Mult0/3(B_re)
  DemuxBim/1 -> Mult0/4(B_im)
  DemuxAre/2 -> Mult1/1(A_re)
  DemuxAim/2 -> Mult1/2(A_im)
  DemuxBre/2 -> Mult1/3(B_re)
  DemuxBim/2 -> Mult1/4(B_im)
  DemuxAre/3 -> Mult2/1(A_re)
  DemuxAim/3 -> Mult2/2(A_im)
  DemuxBre/3 -> Mult2/3(B_re)
  DemuxBim/3 -> Mult2/4(B_im)
  DemuxAre/4 -> Mult3/1(A_re)
  DemuxAim/4 -> Mult3/2(A_im)
  DemuxBre/4 -> Mult3/3(B_re)
  DemuxBim/4 -> Mult3/4(B_im)
  DemuxAre/5 -> Mult4/1(A_re)
  DemuxAim/5 -> Mult4/2(A_im)
  DemuxBre/5 -> Mult4/3(B_re)
  DemuxBim/5 -> Mult4/4(B_im)
  DemuxAre/6 -> Mult5/1(A_re)
  DemuxAim/6 -> Mult5/2(A_im)
  DemuxBre/6 -> Mult5/3(B_re)
  DemuxBim/6 -> Mult5/4(B_im)
  DemuxAre/7 -> Mult6/1(A_re)
  DemuxAim/7 -> Mult6/2(A_im)
  DemuxBre/7 -> Mult6/3(B_re)
  DemuxBim/7 -> Mult6/4(B_im)
  DemuxAre/8 -> Mult7/1(A_re)
  DemuxAim/8 -> Mult7/2(A_im)
  DemuxBre/8 -> Mult7/3(B_re)
  DemuxBim/8 -> Mult7/4(B_im)
  DemuxAre/9 -> Mult8/1(A_re)
  DemuxAim/9 -> Mult8/2(A_im)
  DemuxBre/9 -> Mult8/3(B_re)
  DemuxBim/9 -> Mult8/4(B_im)
  DemuxAre/10 -> Mult9/1(A_re)
  DemuxAim/10 -> Mult9/2(A_im)
  DemuxBre/10 -> Mult9/3(B_re)
  DemuxBim/10 -> Mult9/4(B_im)
  DemuxAre/11 -> Mult10/1(A_re)
  DemuxAim/11 -> Mult10/2(A_im)
  DemuxBre/11 -> Mult10/3(B_re)
  DemuxBim/11 -> Mult10/4(B_im)
  DemuxAre/12 -> Mult11/1(A_re)
  DemuxAim/12 -> Mult11/2(A_im)
  DemuxBre/12 -> Mult11/3(B_re)
  DemuxBim/12 -> Mult11/4(B_im)
  DemuxAre/13 -> Mult12/1(A_re)
  DemuxAim/13 -> Mult12/2(A_im)
  DemuxBre/13 -> Mult12/3(B_re)
  DemuxBim/13 -> Mult12/4(B_im)
  DemuxAre/14 -> Mult13/1(A_re)
  DemuxAim/14 -> Mult13/2(A_im)
  DemuxBre/14 -> Mult13/3(B_re)
  DemuxBim/14 -> Mult13/4(B_im)
  DemuxAre/15 -> Mult14/1(A_re)
  DemuxAim/15 -> Mult14/2(A_im)
  DemuxBre/15 -> Mult14/3(B_re)
  DemuxBim/15 -> Mult14/4(B_im)
  DemuxAre/16 -> Mult15/1(A_re)
  DemuxAim/16 -> Mult15/2(A_im)
  DemuxBre/16 -> Mult15/3(B_re)
  DemuxBim/16 -> Mult15/4(B_im)
  A_re/1 -> DemuxAre/1
  A_im/1 -> DemuxAim/1
  B_re/1 -> DemuxBre/1
  B_im/1 -> DemuxBim/1
